simulink model "Roll_Simulinkpers"  (R2025b)
settings: Solver=VariableStepAuto  StartTime=0.0  StopTime=35  RelTol=1e-3
undefined symbols (not defined in the file): I, rcg_em, rcg_ini, rcg_pr
libraries: aerolibobsolete x1, aerolibatmos2 x1, aerolibnav x1
settings Model: Creator=nitee  LastModifiedBy=niteeshbharadwaj
settings RTWCC: GPUComputeCapability=3.5
settings SimscapeCC: SimscapeLogDataHistory=5000  SimscapeLogDecimation=1

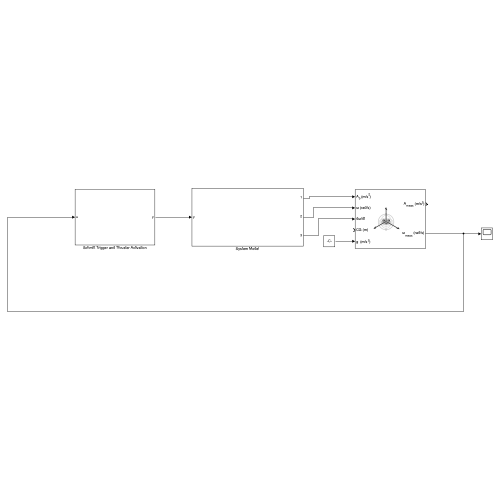
[thumbnail: Simulink's stored preview of the top-level diagram]
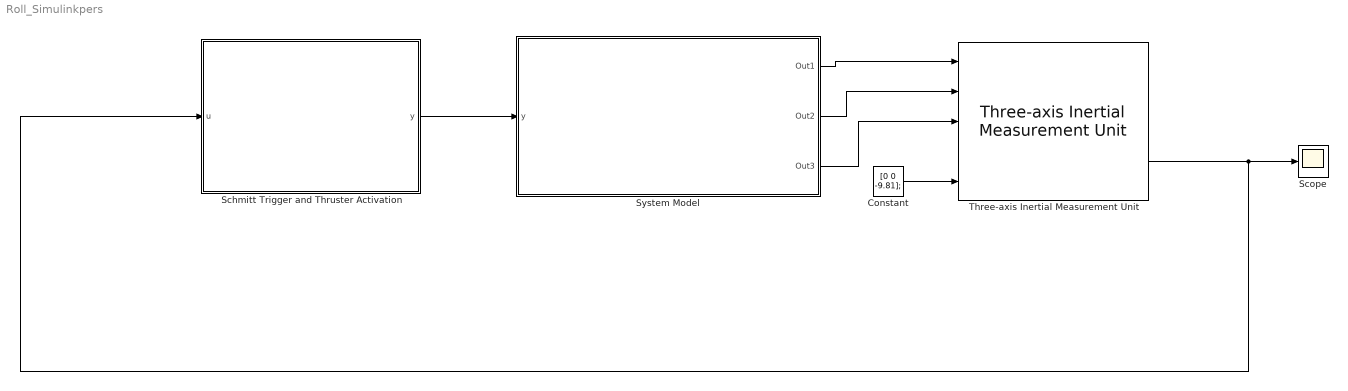
== system Roll_Simulinkpers ==
  Constant : Constant  Value=[0 0 -9.81];
  Schmitt Trigger and Thruster Activation : Subsystem
  Scope : Scope
      settings: ActiveDisplayYMinimum=-512.19994  ActiveDisplayYMaximum=684.51815
  System Model : Subsystem
  Three-axis Inertial Measurement Unit : aerolibnav/Three-axis Inertial Measurement Unit  units=Metric (MKS)  imu=[0 0 0]  i_Ts=0  dtype_a=on  w_a=190  z_a=0.707  a_sf_cc=[1 0 0; 0 1 0; 0 0 1]  a_bias=[0 0 0]  a_sat="[-inf  -inf  -inf  inf inf inf]"  dtype_g=on  w_g=190  z_g=0.707  g_sf_cc=[1 0 0; 0 1 0; 0 0 1]  g_bias=[0 0 0]  g_sens=[0 0 0]  g_sat="[-inf  -inf  -inf  inf inf inf]"  i_rand=on  i_seeds=[23093 23094 23095 23096 23097 23098]  i_pow=[0.001 0.001 0.001 0.0001 0.0001 0.0001]
  wires:
  Three-axis Inertial Measurement Unit/2 -> Scope/1, Schmitt Trigger and Thruster Activation/1(u)
  Schmitt Trigger and Thruster Activation/1(y) -> System Model/1(y)
  System Model/1(Out1) -> Three-axis Inertial Measurement Unit/1
  System Model/2(Out2) -> Three-axis Inertial Measurement Unit/2
  System Model/3(Out3) -> Three-axis Inertial Measurement Unit/3
  Constant/1 -> Three-axis Inertial Measurement Unit/5

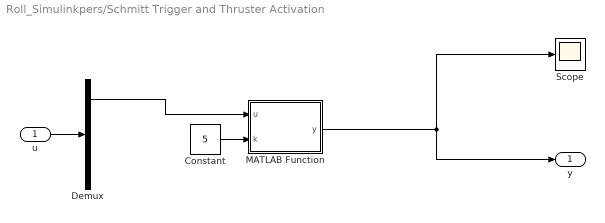
== system Roll_Simulinkpers/Schmitt Trigger and Thruster Activation ==
  u : Inport
  Constant : Constant  Value=5
  Demux : Demux  Outputs=3
  MATLAB Function : MATLAB Function  TreatAsAtomicUnit=on
  Scope : Scope
      settings: ActiveDisplayYMinimum=-1  ActiveDisplayYMaximum=1
  y : Outport
  wires:
  MATLAB Function/1(y) -> Scope/1, y/1
  u/1 -> Demux/1
  Constant/1 -> MATLAB Function/2(k)
  Demux/1 -> MATLAB Function/1(u)

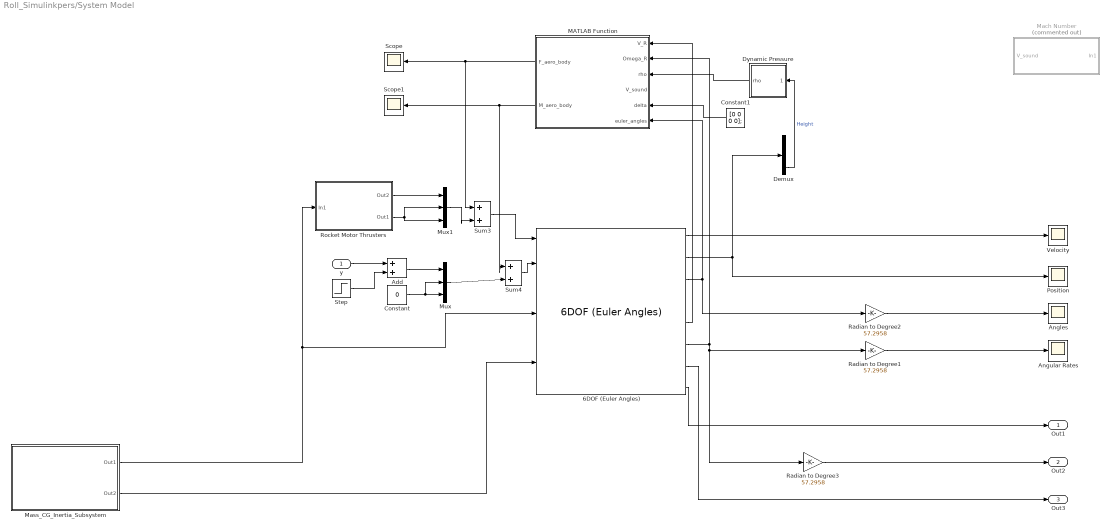
== system Roll_Simulinkpers/System Model ==
  y : Inport
  6DOF (Euler Angles) : aerolibobsolete/6DOF (Euler Angles)  units=Metric (MKS)  mtype=Custom Variable  rep=Euler Angles  xme_0=[0 0 0]  Vm_0=[0 0 0]  eul_0=[0 0 0]  pm_0=[0 0 0]  mass_0=25  mass_e=20  mass_f=25  inertia=eye(3)  inertia_e=eye(3)  inertia_f=2*eye(3)  k_quat=1.0  vre_flag=on  abi_flag=off  aMode=0  xme_statename=''  Vm_statename=''  eul_statename=''  quat_statename=''  pm_statename=''  mass_statename=''
  Add : Sum
  Angles : Scope
      settings: ActiveDisplayYMinimum=-224.95066  ActiveDisplayYMaximum=224.80777  DataLoggingVariableName=ScopeData4
  Angular Rates : Scope
      settings: ActiveDisplayYMinimum=-512.27604  ActiveDisplayYMaximum=685.03419
  Constant : Constant  Value=0
  Constant1 : Constant  Value=[0 0 0 0];
  Demux : Demux  Outputs=3
  Dynamic Pressure : Subsystem
  MATLAB Function : MATLAB Function  TreatAsAtomicUnit=on
  Mach Number : Subsystem  Commented=on
  Mass_CG_Inertia_Subsystem : Subsystem
  Mux : Mux  Inputs=3
  Mux1 : Mux  Inputs=3
  Position : Scope
      settings: ActiveDisplayYMinimum=-131.25002  ActiveDisplayYMaximum=905.94681  DataLoggingVariableName=ScopeData3
  Radian to Degree1 : Gain  Gain=57.2958
  Radian to Degree2 : Gain  Gain=57.2958
  Radian to Degree3 : Gain  Gain=57.2958
  Rocket Motor Thrusters : Subsystem
  Scope : Scope
      settings: ActiveDisplayYMinimum=-1160.96468  ActiveDisplayYMaximum=779.19421
  Scope1 : Scope
      settings: ActiveDisplayYMinimum=-1437.1187  ActiveDisplayYMaximum=1615.36348  DataLoggingVariableName=ScopeData2
  Step : Step  Time=10  Before=0.1  After=0  SampleTime=0
  Sum3 : Sum  Inputs=|++
  Sum4 : Sum  Inputs=|++
  Velocity : Scope
      settings: ActiveDisplayYMinimum=-39.03095  ActiveDisplayYMaximum=134.24121  DataLoggingVariableName=ScopeData2
  Out1 : Outport
  Out2 : Outport  Port=2
  Out3 : Outport  Port=3
  wires:
  Demux/3 -> Dynamic Pressure/1(Height)  "Height"
  Mass_CG_Inertia_Subsystem/1(Out1) -> Rocket Motor Thrusters/1(In1), 6DOF (Euler Angles)/4
  Mass_CG_Inertia_Subsystem/2(Out2) -> 6DOF (Euler Angles)/6
  Mux1/1 -> Sum3/2
  6DOF (Euler Angles)/5 -> MATLAB Function/1(V_R)
  6DOF (Euler Angles)/2 -> Position/1, Demux/1
  Mux/1 -> Sum4/2
  Sum4/1 -> 6DOF (Euler Angles)/2
  Sum3/1 -> 6DOF (Euler Angles)/1
  6DOF (Euler Angles)/6 -> Radian to Degree3/1, Radian to Degree1/1, MATLAB Function/2(Omega_R)
  6DOF (Euler Angles)/3 -> MATLAB Function/6(euler_angles), Radian to Degree2/1
  6DOF (Euler Angles)/1 -> Velocity/1
  Radian to Degree1/1 -> Angular Rates/1
  y/1 -> Add/1
  Step/1 -> Add/2
  Radian to Degree2/1 -> Angles/1
  Constant1/1 -> MATLAB Function/5(delta)
  Dynamic Pressure/1(rho) -> MATLAB Function/3(rho)
  MATLAB Function/1(F_aero_body) -> Scope/1, Sum3/1
  MATLAB Function/2(M_aero_body) -> Sum4/1, Scope1/1
  Rocket Motor Thrusters/1(Out2) -> Mux1/1
  Rocket Motor Thrusters/2(Out1) -> Mux1/2, Mux1/3
  Constant/1 -> Mux/2, Mux/3
  Add/1 -> Mux/1
  6DOF (Euler Angles)/8 -> Out1/1
  Radian to Degree3/1 -> Out2/1
  6DOF (Euler Angles)/7 -> Out3/1

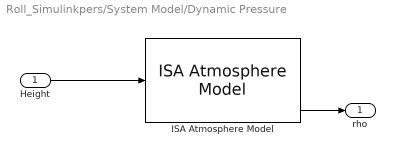
== system Roll_Simulinkpers/System Model/Dynamic Pressure ==
  Height : Inport
  ISA Atmosphere Model : aerolibatmos2/ISA Atmosphere Model  useExtended=off  action=Warning  custom=off  viscosityOut=off  g=9.80665  gamma=1.4  R=287.0531  L=0.0065  h_trop=11000  h_strat=20000  rho0=1.225  P0=101325  T0=288.15  h0=0
  rho : Outport
  wires:
  Height/1 -> ISA Atmosphere Model/1
  ISA Atmosphere Model/4 -> rho/1

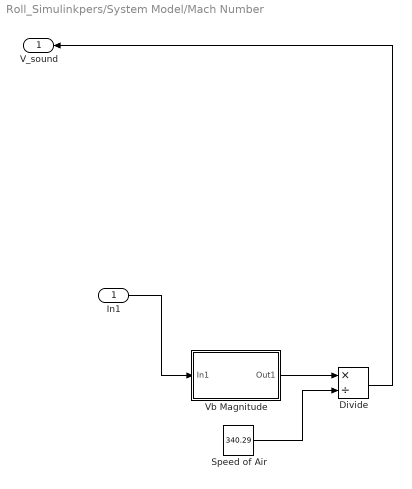
== system Roll_Simulinkpers/System Model/Mach Number ==
  In1 : Inport
  Divide : Product  Inputs=*/
  Speed of Air : Constant  Value=340.29
  Vb Magnitude : Subsystem
  V_sound : Outport
  wires:
  Vb Magnitude/1(Out1) -> Divide/1
  Speed of Air/1 -> Divide/2
  In1/1 -> Vb Magnitude/1(In1)
  Divide/1 -> V_sound/1

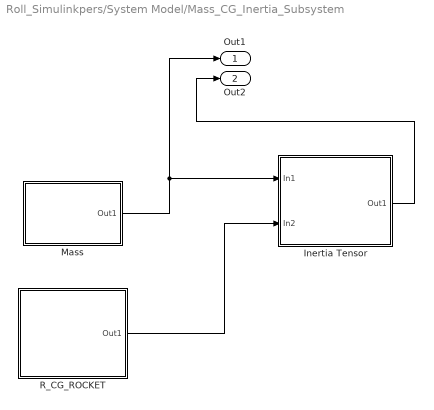
== system Roll_Simulinkpers/System Model/Mass_CG_Inertia_Subsystem ==
  "Inertia Tensor " : Subsystem
  Mass : Subsystem
  R_CG_ROCKET : Subsystem
  Out1 : Outport
  Out2 : Outport  Port=2
  wires:
  Mass/1(Out1) -> Out1/1, "Inertia Tensor "/1(In1)
  R_CG_ROCKET/1(Out1) -> "Inertia Tensor "/2(In2)
  "Inertia Tensor "/1(Out1) -> Out2/1

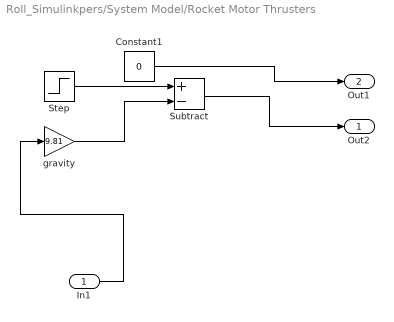
== system Roll_Simulinkpers/System Model/Rocket Motor Thrusters ==
  In1 : Inport
  Constant1 : Constant  Value=0
  Step : Step  Time=5  Before=800  After=0  SampleTime=0
  Subtract : Sum  Inputs=+-
  gravity : Gain  Gain=9.81
  Out2 : Outport
  Out1 : Outport  Port=2
  wires:
  In1/1 -> gravity/1
  gravity/1 -> Subtract/2
  Step/1 -> Subtract/1
  Subtract/1 -> Out2/1
  Constant1/1 -> Out1/1

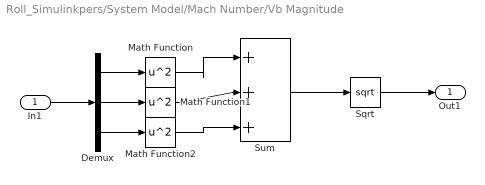
== system Roll_Simulinkpers/System Model/Mach Number/Vb Magnitude ==
  In1 : Inport
  Demux : Demux  Outputs=3
  Math Function : Math  Operator=square
  Math Function1 : Math  Operator=square
  Math Function2 : Math  Operator=square
  Sqrt : Sqrt
  Sum : Sum  Inputs=|+++
  Out1 : Outport
  wires:
  In1/1 -> Demux/1
  Demux/1 -> Math Function/1
  Demux/3 -> Math Function2/1
  Math Function/1 -> Sum/1
  Math Function2/1 -> Sum/3
  Sum/1 -> Sqrt/1
  Sqrt/1 -> Out1/1
  Demux/2 -> Math Function1/1
  Math Function1/1 -> Sum/2

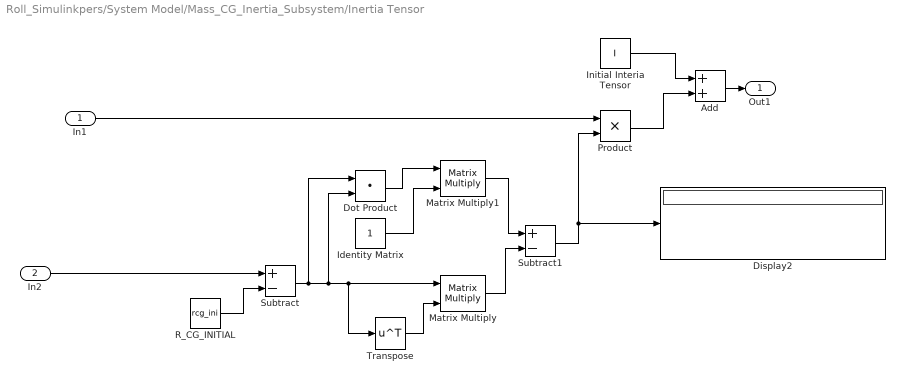
== system Roll_Simulinkpers/System Model/Mass_CG_Inertia_Subsystem/Inertia Tensor  ==
  In1 : Inport
  In2 : Inport  Port=2
  Add : Sum
  Display2 : Display
  Dot Product : DotProduct  OutDataTypeStr=Inherit: Inherit via internal rule
  Identity Matrix : Constant
  Initial Interia Tensor : Constant  Value=I
  Matrix Multiply : Product  Multiplication=Matrix(*)
  Matrix Multiply1 : Product  Multiplication=Matrix(*)
  Product : Product
  R_CG_INITIAL : Constant  Value=rcg_ini
  Subtract : Sum  Inputs=+-
  Subtract1 : Sum  Inputs=+-
  Transpose : Math  Operator=transpose
  Out1 : Outport
  wires:
  Subtract1/1 -> Product/2, Display2/1
  Subtract/1 -> Dot Product/1, Dot Product/2, Matrix Multiply/1, Transpose/1
  Add/1 -> Out1/1
  Transpose/1 -> Matrix Multiply/2
  Dot Product/1 -> Matrix Multiply1/1
  Product/1 -> Add/2
  R_CG_INITIAL/1 -> Subtract/2
  Initial Interia Tensor/1 -> Add/1
  Identity Matrix/1 -> Matrix Multiply1/2
  Matrix Multiply1/1 -> Subtract1/1
  Matrix Multiply/1 -> Subtract1/2
  In1/1 -> Product/1
  In2/1 -> Subtract/1

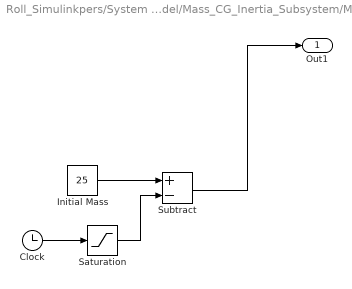
== system Roll_Simulinkpers/System Model/Mass_CG_Inertia_Subsystem/Mass ==
  Clock : Clock
  Initial Mass : Constant  Value=25
  Saturation : Saturate  UpperLimit=5  LowerLimit=0
  Subtract : Sum  Inputs=+-
  Out1 : Outport
  wires:
  Subtract/1 -> Out1/1
  Initial Mass/1 -> Subtract/1
  Clock/1 -> Saturation/1
  Saturation/1 -> Subtract/2

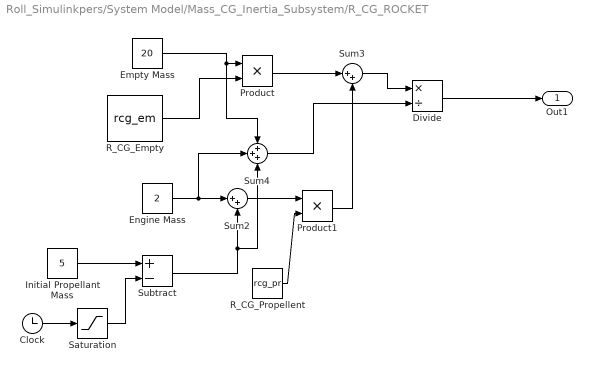
== system Roll_Simulinkpers/System Model/Mass_CG_Inertia_Subsystem/R_CG_ROCKET ==
  Clock : Clock
  Divide : Product  Inputs=*/
  Empty Mass : Constant  Value=20
  Engine Mass : Constant  Value=2
  Initial Propellant Mass : Constant  Value=5
  Product : Product
  Product1 : Product
  R_CG_Empty : Constant  Value=rcg_em
  R_CG_Propellent : Constant  Value=rcg_pr
  Saturation : Saturate  UpperLimit=5  LowerLimit=0
  Subtract : Sum  Inputs=+-
  Sum2 : Sum  Inputs=|++
  Sum3 : Sum  Inputs=|++
  Sum4 : Sum  Inputs=+++
  Out1 : Outport
  wires:
  Divide/1 -> Out1/1
  Sum4/1 -> Divide/2
  Engine Mass/1 -> Sum4/2, Sum2/1
  Sum3/1 -> Divide/1
  R_CG_Propellent/1 -> Product1/2
  Empty Mass/1 -> Sum4/1, Product/1
  Subtract/1 -> Sum4/3, Sum2/2
  R_CG_Empty/1 -> Product/2
  Sum2/1 -> Product1/1
  Product/1 -> Sum3/1
  Product1/1 -> Sum3/2
  Initial Propellant Mass/1 -> Subtract/1
  Clock/1 -> Saturation/1
  Saturation/1 -> Subtract/2

== matlab function Roll_Simulinkpers/System Model/MATLAB Function ==
  data: V_R input; F_aero_body output; Omega_R input; rho input; V_sound input; delta input; M_aero_body output; euler_angles input
function [F_aero_body, M_aero_body] = aerodynamic_model(V_R, Omega_R, rho, V_sound, delta, euler_angles)
% AERODYNAMIC_MODEL Calculates aerodynamic forces and moments for the GENESYS rocket.
%
% UPDATE: Added logic to rotate the body-frame forces into the Earth-fixed frame.
%
% Inputs:
%   V_R          - 3x1 vector of velocity in the body frame [u, v, w] (m/s)
%   Omega_R      - 3x1 vector of angular rates in the body frame [p, q, r] (rad/s)
%   rho          - Scalar, air density at current altitude (kg/m^3)
%   V_sound      - Scalar, speed of sound at current altitude (m/s)
%   delta        - 4x1 vector of fin misalignment angles [d1, d2, d3, d4] (rad)
%   euler_angles - 3x1 vector of attitude [roll, pitch, yaw] or [phi, theta, psi] (rad)
%
% Outputs:
%   F_aero_body  - 3x1 vector of aerodynamic forces in the BODY frame [X, Y, Z] (N)
%   M_aero_body  - 3x1 vector of aerodynamic moments in the BODY frame [l, m, n] (Nm)
%   F_aero_earth - 3x1 vector of aerodynamic forces in the EARTH frame [Fx, Fy, Fz] (N)
%   q_bar_out    - Scalar, calculated dynamic pressure (Pa) for diagnostics.

% --- Section 1: Define Rocket Geometric and Aerodynamic Constants ---
A_ref = 0.0491;     % Reference Area (m^2)
d = 0.25;           % Rocket Diameter (m)
C_X0 = 0.3869;      
k_ail = 7.5620;     
C_Y0 = -0.0167;     
C_Y_beta = 17.3995; 
C_Z0 = -0.0263;     
C_Z_alpha = 17.3395;
C_lp = -49.3811;    
C_m0 = 0.2447;      
C_m_alpha = -144.7088; 
C_mq = -1497.6;     
C_n0 = -0.1554;     
C_n_beta = 144.7088;  
C_nr = -1497.6;     
Rc = 0.238; 
C_Z_alpha_ail = 2.76; 

% --- Section 2: Calculate Current Flight Conditions ---
u = V_R(1); 
v = V_R(2); 
w = V_R(3);
p = Omega_R(1); 
q = Omega_R(2); 
r = Omega_R(3);

V = norm(V_R);
if V < 1e-6 
    V = 1e-6;
end

alpha = atan2(w, u);
beta = asin(v / V);
q_bar = 0.5 * rho * V^2;

% --- Section 3: Calculate Aerodynamic Forces in Body Frame ---
C_Xi = k_ail * ( (alpha + delta(3) + delta(4))^2 + (beta + delta(1) + delta(2))^2 );
C_X = C_X0 + C_Xi;
C_Y = C_Y0 + C_Y_beta * beta;
C_Z = C_Z0 + C_Z_alpha * alpha;

X_body = -q_bar * A_ref * C_X;
Y_body =  q_bar * A_ref * C_Y;
Z_body =  q_bar * A_ref * C_Z;

F_aero_body = [X_body; Y_body; Z_body];

% --- Section 4: Calculate Aerodynamic Moments in Body Frame ---
p_hat = p * d / (2 * V);
q_hat = q * d / (2 * V);
r_hat = r * d / (2 * V);

C_l0_dynamic = C_Z_alpha_ail * (delta(1) - delta(2) + delta(3) - delta(4)) * (Rc / d);
C_l = C_l0_dynamic + C_lp * p_hat;
C_m = C_m0 + C_m_alpha * alpha + C_mq * q_hat;
C_n = C_n0 + C_n_beta * beta + C_nr * r_hat;

l_body = q_bar * A_ref * d * C_l;
m_body = q_bar * A_ref * d * C_m;
n_body = q_bar * A_ref * d * C_n;

M_aero_body = [l_body; m_body; n_body];

end

== matlab function Roll_Simulinkpers/Schmitt Trigger and Thruster Activation/MATLAB Function ==
  data: u input; y output; k input
function y = fcn(u, k)
% FCN Implements a thruster controller with a deadband.
%
% This function models a thruster's behavior based on an angular rate 'u'.
% It includes a deadband between -5 and 5, where no thruster is activated.
%
% Logic:
% - If u is greater than 5, the thruster provides -30N of force.
% - If u is less than -5, the thruster provides 30N of force.
% - If u is between -5 and 5 (inclusive), the thruster is off (0N).
%
% Input:
%   u - The input angular rate (can be a scalar or a vector).
%
% Output:
%   y - The thruster output (30, -30, or 0).

    % This vectorized expression calculates the output in a single line.
    % It evaluates two logical conditions:
    % 1. (u < -5): Returns 1 if true, 0 otherwise. This is multiplied by 30.
    % 2. (u > 5):  Returns 1 if true, 0 otherwise. This is multiplied by -30.
    % If 'u' is in the deadband, both conditions are false, resulting in an
    % output of 0. Otherwise, only one condition can be true, yielding
    % either 30 or -30.
    y = (10 * (u < -k)) + (-10 * (u > k));
    
end
